simulink model "Pacemaker"  (R2020a)
settings: Solver=FixedStepAuto  StartTime=0.0  StopTime=10.0  FixedStep=1e-3  RelTol=1e-3  EnableMultiTasking=on
InitFcn:
  | ATR_SENSING = Simulink.Variant('Sensed == 1');
  | VENT_SENSING = Simulink.Variant('Sensed == 2');
  | Sensed = 2;
  | 
  | O_RESPONSE = Simulink.Variant('Response == 1');
  | I_RESPONSE = Simulink.Variant('Response == 2');
  | Response = 2;
  | 
  | ATR_PACING = Simulink.Variant('Paced == 1');
  | VENT_PACING = Simulink.Variant('Paced == 2');
  | DUAL_PACING = Simulink.Variant('Paced == 3');
  | Paced = 2;
libraries: frdmk64flib x2
settings Model: ExtModeTrigDuration=5  Creator=WinnieTrandinh  LastModifiedBy=WinnieTrandinh
settings OptimizationCC: EnhancedBackFolding=on  PassReuseOutputArgsAs=Individual arguments  ZeroExternalMemoryAtStartup=off  ZeroInternalMemoryAtStartup=off  MaxStackSize=64  OptimizeBlockOrder=speed  DifferentSizesBufferReuse=on  OptimizationCustomize=off  EfficientTunableParamExpr=on
settings DebuggingCC: ParameterTunabilityLossMsg=error
settings HardwareCC: ProdBitPerPointer=32  ProdBitPerSizeT=32  ProdBitPerPtrDiffT=32  ProdLargestAtomicInteger=Long  ProdLargestAtomicFloat=Double  ProdWordSize=32  ProdHWDeviceType=ARM Compatible->ARM Cortex
settings SFSimCC: MATLABDynamicMemAlloc=off
settings RTWCC: SystemTargetFile=ert.tlc  HardwareBoard=NXP FRDM-K64F  TemplateMakefile=ert_default_tmf  Toolchain=GNU Tools for ARM Embedded Processors
settings CodeAppCC: ForceParamTrailComments=on  IgnoreCustomStorageClasses=off  OperatorAnnotations=on  SimulinkDataObjDesc=on  SFDataObjDesc=on  InsertBlockDesc=on

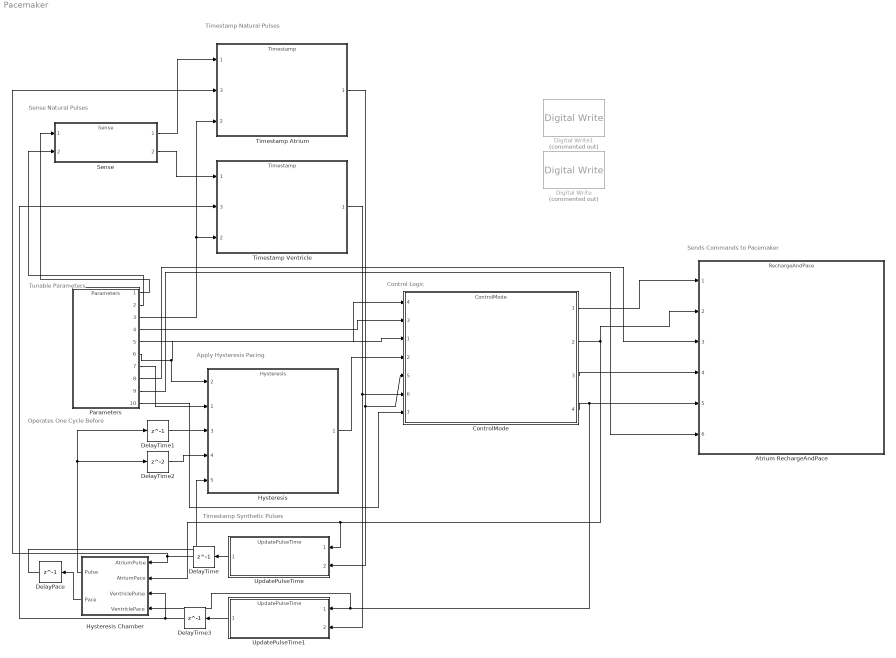
== system Pacemaker ==
  note: Sends Commands to Pacemaker
  note: Control Logic
  note: Timestamp Natural Pulses
  note: Sense Natural Pulses
  note: Timestamp Synthetic Pulses
  note: Apply Hysteresis Pacing
  note: Operates One Cycle Before
  note: Tunable
      | Parameters
  Atrium RechargeAndPace : ModelReference  ModelNameDialog=RechargeAndPace.slx  SimulationMode=Normal  ModelReferenceVersion=1.43
  ControlMode : ModelReference  ModelNameDialog=ControlMode.slx  SimulationMode=Normal  ModelReferenceVersion=1.22
      settings: PortSchema="{\"entries\":[{\"content\":{\"sides\":[{\"content\":{\"connectorIds\":[\"In4\",\"In3\",\"In1\",\"In2\",\"In5\",\"In6\",\"In7\"]},\"type\":\"ConnectorPlacement.EquallySpacedRectSide\",\"uuid\":\"6632d3f0-aa64-4d08-bbe9-86261208e7ec\"},{\"content\":{\"connectorIds\":[\"Out1\",\"Out2\",\"Out3\",\"Out4\"],\"side\":\"RIGHT\"},\"type\":\"ConnectorPlacement.EquallySpacedRectSide\",\"uuid\":\"64c7d09c-149d-4c40-8331-deac9c0e6c2d\"},{\"content\":{\"connectorIds\":[],\"side\":\"TOP\"},\"type\":\"ConnectorPlacement.EquallySpacedRectSide\",\"uuid\":\"acc88ae8-e334-42c0-8332-b39c537b29da\"}]},\"type\":\"ConnectorPlacement.EquallySpacedConnector\",\"uuid\":\"2c09cc21-dcc5-4040-85e7-e7c3f2d085fd\"}],\"packageUris\":[\"http://schema.mathworks.com/mf0/Connector/19700101\"],\"version\":\"1.0\"}"
  DelayPace : Delay  DelayLength=1
  DelayTime : Delay  DelayLength=1
  DelayTime1 : Delay  DelayLength=1
  DelayTime2 : Delay
  DelayTime3 : Delay  DelayLength=1
  Digital Write : frdmk64flib/Digital Write  Commented=on  Whichpin=GREEN_LED
  Digital Write1 : frdmk64flib/Digital Write  Commented=on  Whichpin=BLUE_LED
  Hysteresis : ModelReference  ModelNameDialog=Hysteresis.slx  SimulationMode=Normal  ModelReferenceVersion=1.20
      settings: PortSchema="{\"entries\":[{\"content\":{\"sides\":[{\"content\":{\"connectorIds\":[\"In2\",\"In1\",\"In3\",\"In4\",\"In5\"]},\"type\":\"ConnectorPlacement.EquallySpacedRectSide\",\"uuid\":\"0363428c-2bcd-4f6e-9e7c-a7a2e1284dda\"},{\"content\":{\"connectorIds\":[\"Out1\"],\"side\":\"RIGHT\"},\"type\":\"ConnectorPlacement.EquallySpacedRectSide\",\"uuid\":\"eba4b486-06a8-42d4-b87a-2bd50947fa00\"},{\"content\":{\"connectorIds\":[],\"side\":\"TOP\"},\"type\":\"ConnectorPlacement.EquallySpacedRectSide\",\"uuid\":\"d7235661-47f4-47cb-815b-72bf3af657d3\"}]},\"type\":\"ConnectorPlacement.EquallySpacedConnector\",\"uuid\":\"f6a939f5-0e90-4bb6-9df3-6cabec2ca3b5\"}],\"packageUris\":[\"http://schema.mathworks.com/mf0/Connector/19700101\"],\"version\":\"1.0\"}"
  Hysteresis Chamber : Subsystem  Variant=on
  Parameters : ModelReference  ModelNameDialog=Parameters.slx  SimulationMode=Normal  ModelReferenceVersion=1.2
  Sense : ModelReference  ModelNameDialog=Sense.slx  SimulationMode=Normal  ModelReferenceVersion=1.33
  Timestamp Atrium : ModelReference  ModelNameDialog=Timestamp.slx  SimulationMode=Normal  ModelReferenceVersion=1.20
      settings: PortSchema="{\"entries\":[{\"content\":{\"sides\":[{\"content\":{\"connectorIds\":[\"In1\",\"In3\",\"In2\"]},\"type\":\"ConnectorPlacement.EquallySpacedRectSide\",\"uuid\":\"07fba71a-3d16-4041-80f3-8d8caa2e5429\"},{\"content\":{\"connectorIds\":[\"Out1\"],\"side\":\"RIGHT\"},\"type\":\"ConnectorPlacement.EquallySpacedRectSide\",\"uuid\":\"c6e0a25f-6fc6-4904-ad60-49887298795d\"},{\"content\":{\"connectorIds\":[],\"side\":\"TOP\"},\"type\":\"ConnectorPlacement.EquallySpacedRectSide\",\"uuid\":\"2ac2bd4a-2ab8-4c90-9fc4-ba83a2e83542\"}]},\"type\":\"ConnectorPlacement.EquallySpacedConnector\",\"uuid\":\"9f017194-9fcb-4cde-9b1c-0209ce44303b\"}],\"packageUris\":[\"http://schema.mathworks.com/mf0/Connector/19700101\"],\"version\":\"1.0\"}"
  Timestamp Ventricle : ModelReference  ModelNameDialog=Timestamp.slx  SimulationMode=Normal  ModelReferenceVersion=1.20
      settings: PortSchema="{\"entries\":[{\"content\":{\"sides\":[{\"content\":{\"connectorIds\":[\"In1\",\"In3\",\"In2\"]},\"type\":\"ConnectorPlacement.EquallySpacedRectSide\",\"uuid\":\"07fba71a-3d16-4041-80f3-8d8caa2e5429\"},{\"content\":{\"connectorIds\":[\"Out1\"],\"side\":\"RIGHT\"},\"type\":\"ConnectorPlacement.EquallySpacedRectSide\",\"uuid\":\"c6e0a25f-6fc6-4904-ad60-49887298795d\"},{\"content\":{\"connectorIds\":[],\"side\":\"TOP\"},\"type\":\"ConnectorPlacement.EquallySpacedRectSide\",\"uuid\":\"2ac2bd4a-2ab8-4c90-9fc4-ba83a2e83542\"}]},\"type\":\"ConnectorPlacement.EquallySpacedConnector\",\"uuid\":\"9f017194-9fcb-4cde-9b1c-0209ce44303b\"}],\"packageUris\":[\"http://schema.mathworks.com/mf0/Connector/19700101\"],\"version\":\"1.0\"}"
  UpdatePulseTime : ModelReference  ModelNameDialog=UpdatePulseTime.slx  SimulationMode=Normal  ModelReferenceVersion=1.13
  UpdatePulseTime1 : ModelReference  ModelNameDialog=UpdatePulseTime.slx  SimulationMode=Normal  ModelReferenceVersion=1.13
  wires:
  Sense/1 -> Timestamp Atrium/1
  Timestamp Atrium/1 -> ControlMode/5, UpdatePulseTime/2
  ControlMode/1 -> Atrium RechargeAndPace/1
  ControlMode/2 -> Hysteresis Chamber/2(AtriumPace), UpdatePulseTime/1, Atrium RechargeAndPace/2
  DelayTime2/1 -> Hysteresis/4
  DelayPace/1 -> Hysteresis/5
  DelayTime1/1 -> Hysteresis/3
  Hysteresis/1 -> ControlMode/2
  Parameters/6 -> Hysteresis/2, ControlMode/1
  Parameters/7 -> Hysteresis/1
  Parameters/3 -> Timestamp Ventricle/2, Timestamp Atrium/2
  Parameters/1 -> Sense/1
  Parameters/2 -> Sense/2
  Parameters/4 -> ControlMode/3
  Parameters/5 -> ControlMode/4
  Parameters/8 -> Atrium RechargeAndPace/3
  Sense/2 -> Timestamp Ventricle/1
  Timestamp Ventricle/1 -> UpdatePulseTime1/2, ControlMode/6
  ControlMode/4 -> Atrium RechargeAndPace/5, Hysteresis Chamber/4(VentriclePace), UpdatePulseTime1/1
  Hysteresis Chamber/2(Pace) -> DelayPace/1
  UpdatePulseTime/1 -> DelayTime/1
  DelayTime/1 -> Timestamp Atrium/3, Hysteresis Chamber/1(AtriumPulse)
  UpdatePulseTime1/1 -> DelayTime3/1
  DelayTime3/1 -> Timestamp Ventricle/3, Hysteresis Chamber/3(VentriclePulse)
  Hysteresis Chamber/1(Pulse) -> DelayTime1/1, DelayTime2/1
  ControlMode/3 -> Atrium RechargeAndPace/4
  Parameters/9 -> Atrium RechargeAndPace/6
  Parameters/10 -> ControlMode/7

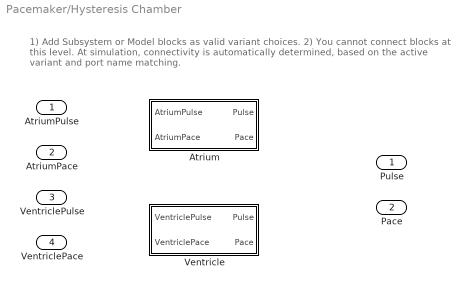
== system Pacemaker/Hysteresis Chamber ==
  note: 1) Add Subsystem or Model blocks as valid variant choices.
      | 2) You cannot connect blocks at this level. At simulation, connectivity is automatically
      | determined, based on the active variant and port name matching.
  AtriumPulse : Inport
  AtriumPace : Inport  Port=2
  VentriclePulse : Inport  Port=3
  VentriclePace : Inport  Port=4
  Atrium : Subsystem  VariantControl=ATR_SENSING
  Ventricle : Subsystem  VariantControl=VENT_SENSING
  Pulse : Outport
  Pace : Outport  Port=2

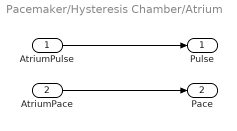
== system Pacemaker/Hysteresis Chamber/Atrium ==
  AtriumPulse : Inport
  AtriumPace : Inport  Port=2
  Pulse : Outport
  Pace : Outport  Port=2
  wires:
  AtriumPulse/1 -> Pulse/1
  AtriumPace/1 -> Pace/1

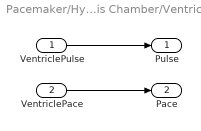
== system Pacemaker/Hysteresis Chamber/Ventricle ==
  VentriclePulse : Inport
  VentriclePace : Inport  Port=2
  Pulse : Outport
  Pace : Outport  Port=2
  wires:
  VentriclePulse/1 -> Pulse/1
  VentriclePace/1 -> Pace/1
